simulink model "day04"  (R2026a)
settings: Solver=VariableStepAuto  StopTime=inf
libraries: simulink x1
settings Model: Creator=pete  LastModifiedBy=pete

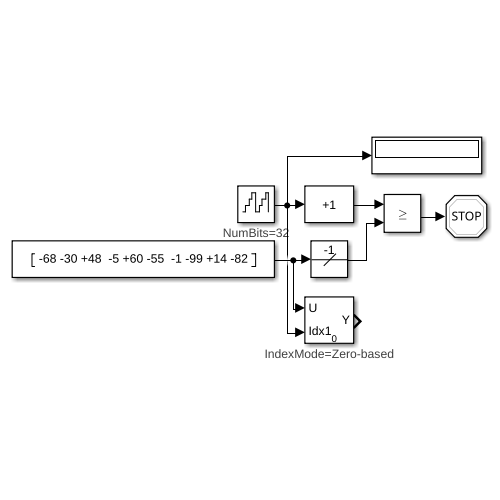
[thumbnail: Simulink's stored preview of the top-level diagram]
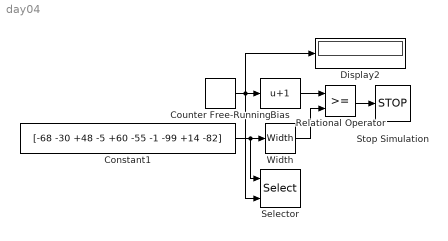
== system day04 ==
  Bias : Bias  Bias=1  SaturateOnIntegerOverflow=off
  Constant1 : Constant  Value=[-68 -30 +48 -5 +60 -55 -1 -99 +14 -82]
  Counter Free-Running : simulink/Sources/Counter Free-Running  NumBits=32  tsamp=-1
      settings: AttributesFormatString=NumBits=%<NumBits>
  Display2 : Display
  Relational Operator : RelationalOperator  OutDataTypeStr=boolean  RndMeth=Simplest  InputSameDT=off
  Selector : Selector  IndexMode=Zero-based  InputPortWidth=10  IndexOptions=Index vector (port)  Indices=[1 3]  OutputSizes=1
      settings: AttributesFormatString=IndexMode=%<IndexMode>
  Stop Simulation : Stop
  Width : Width
  wires:
  Counter Free-Running/1 -> Display2/1, Selector/2, Bias/1
  Bias/1 -> Relational Operator/1
  Relational Operator/1 -> Stop Simulation/1
  Width/1 -> Relational Operator/2
  Constant1/1 -> Selector/1, Width/1
